simulink subsystem "Vwilly2Vcartesiana"  (R2021b)
settings: Solver=VariableStepAuto  StartTime=0.0  StopTime=10.0  RelTol=1e-3
settings Model: Creator=Mauri  LastModifiedBy=Mauri

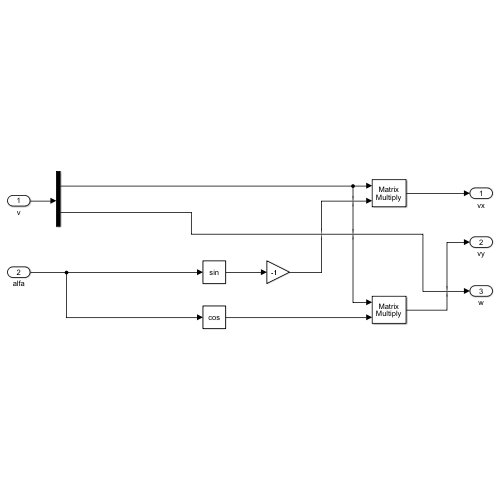
[thumbnail: Simulink's stored preview of the top-level diagram]
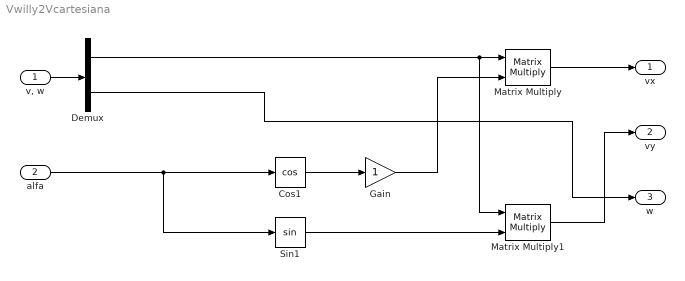
== system Vwilly2Vcartesiana ==
  "v, w" : Inport
  alfa : Inport  Port=2
  Cos1 : Trigonometry  Operator=cos
  Demux : Demux  Outputs=2
  Gain : Gain
  Matrix Multiply : Product  Multiplication=Matrix(*)
  Matrix Multiply1 : Product  Multiplication=Matrix(*)
  Sin1 : Trigonometry
  vx : Outport
  vy : Outport  Port=2
  w : Outport  Port=3
  wires:
  Matrix Multiply1/1 -> vy/1
  Matrix Multiply/1 -> vx/1
  Demux/2 -> w/1
  Gain/1 -> Matrix Multiply/2
  Demux/1 -> Matrix Multiply/1, Matrix Multiply1/1
  Cos1/1 -> Gain/1
  alfa/1 -> Sin1/1, Cos1/1
  "v, w"/1 -> Demux/1
  Sin1/1 -> Matrix Multiply1/2
